simulink model "CyberDog_Motor_FOC_Test"  (R2025b)
settings: Solver=ode4  StartTime=0.0  StopTime=5  FixedStep=0.0001  RelTol=1e-3
InitFcn:
  | p = fileparts(get_param(bdroot,'FileName')); addpath(fullfile(p,'scripts')); motor_params;
undefined symbols (not defined in the file): PolePairs_plant, T_ctrl_mode, T_iq_ref, T_ref_speed, T_TL, Vbus_plant
libraries: mcbplantlib x1, autolibpmsmexterior x1
settings Model: Creator=Baseline  LastModifiedBy=Baseline

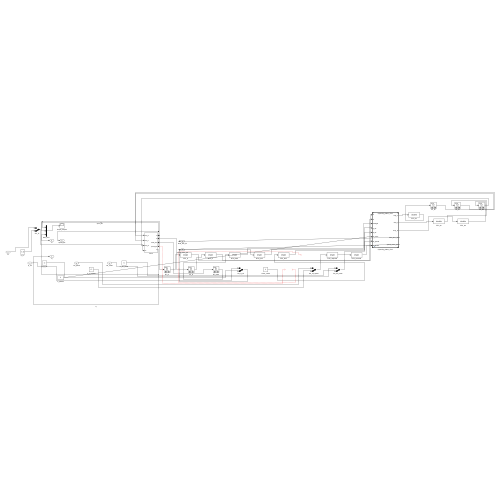
[thumbnail: Simulink's stored preview of the top-level diagram]
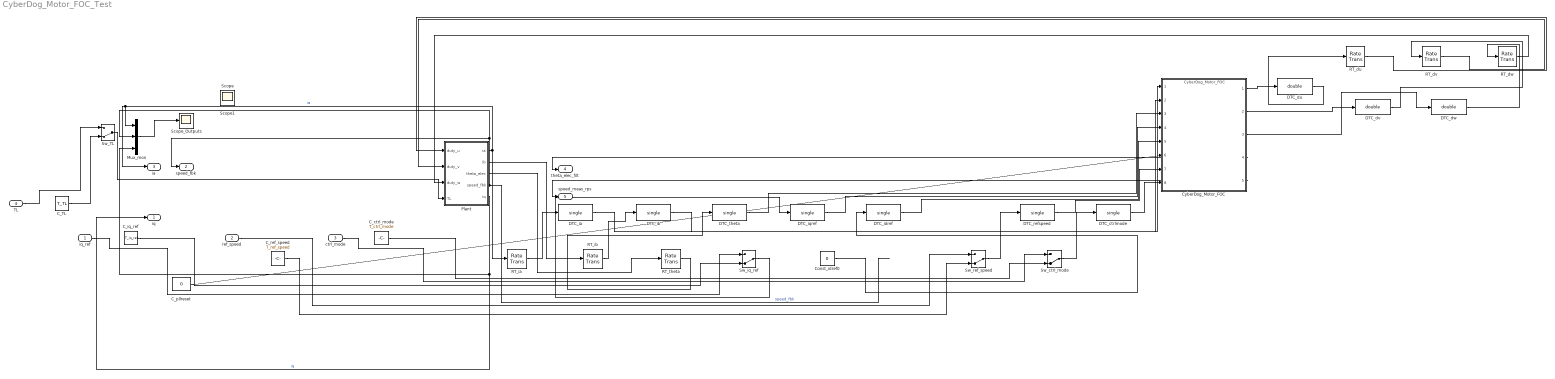
== system CyberDog_Motor_FOC_Test ==
  iq_ref : Inport
  ref_speed : Inport  Port=2
  ctrl_mode : Inport  Port=3
  TL : Inport  Port=4
  C_TL : Constant  Value=T_TL
  C_ctrl_mode : Constant  Value=T_ctrl_mode
  C_iq_ref : Constant  Value=T_iq_ref
  C_pllreset : Constant  Value=0  OutDataTypeStr=single
  C_ref_speed : Constant  Value=T_ref_speed
  Const_idref0 : Constant  Value=0
  CyberDog_Motor_FOC : ModelReference  ModelNameDialog=CyberDog_Motor_FOC  SimulationMode=Normal  ModelReferenceVersion=1.26
  DTC_ctrlmode : DataTypeConversion  OutDataTypeStr=single  SaturateOnIntegerOverflow=off  RndMeth=Floor
  DTC_du : DataTypeConversion  OutDataTypeStr=double  SaturateOnIntegerOverflow=off  RndMeth=Floor
  DTC_dv : DataTypeConversion  OutDataTypeStr=double  SaturateOnIntegerOverflow=off  RndMeth=Floor
  DTC_dw : DataTypeConversion  OutDataTypeStr=double  SaturateOnIntegerOverflow=off  RndMeth=Floor
  DTC_ia : DataTypeConversion  OutDataTypeStr=single  SaturateOnIntegerOverflow=off  RndMeth=Floor
  DTC_ib : DataTypeConversion  OutDataTypeStr=single  SaturateOnIntegerOverflow=off  RndMeth=Floor
  DTC_idref : DataTypeConversion  OutDataTypeStr=single  SaturateOnIntegerOverflow=off  RndMeth=Floor
  DTC_iqref : DataTypeConversion  OutDataTypeStr=single  SaturateOnIntegerOverflow=off  RndMeth=Floor
  DTC_refspeed : DataTypeConversion  OutDataTypeStr=single  SaturateOnIntegerOverflow=off  RndMeth=Floor
  DTC_theta : DataTypeConversion  OutDataTypeStr=single  SaturateOnIntegerOverflow=off  RndMeth=Floor
  Mux_mon : Mux  Inputs=3
  Plant : Subsystem
  RT_du : RateTransition
  RT_dv : RateTransition
  RT_dw : RateTransition
  RT_ia : RateTransition
  RT_ib : RateTransition
  RT_theta : RateTransition
  Scope_Outputs : Scope
      settings: ActiveDisplayYMinimum=-11.406382448656982  ActiveDisplayYMaximum=18.168654247601083
  Sw_TL : ManualSwitch  CurrentSetting=0
  Sw_ctrl_mode : ManualSwitch  CurrentSetting=0
  Sw_iq_ref : ManualSwitch  CurrentSetting=0
  Sw_ref_speed : ManualSwitch  CurrentSetting=0
  iq : Outport
  speed_fbk : Outport  Port=2
  ia : Outport  Port=3
  theta_elec_filt : Outport  Port=4
  speed_meas_rps : Outport  Port=5
  Scope : Scope
      settings: ActiveDisplayYMinimum=-1  ActiveDisplayYMaximum=1
  Scope1 : Scope
      settings: ActiveDisplayYMinimum=-1  ActiveDisplayYMaximum=1
  wires:
  C_TL/1 -> Sw_TL/2
  TL/1 -> Sw_TL/1
  Mux_mon/1 -> Scope_Outputs/1
  Sw_TL/1 -> Plant/4(TL)
  Plant/5(iq) -> iq/1, Mux_mon/3  "iq"
  DTC_dw/1 -> RT_dw/1
  DTC_dv/1 -> RT_dv/1
  DTC_du/1 -> RT_du/1
  DTC_ctrlmode/1 -> CyberDog_Motor_FOC/8
  DTC_refspeed/1 -> CyberDog_Motor_FOC/7
  DTC_idref/1 -> CyberDog_Motor_FOC/5
  DTC_iqref/1 -> CyberDog_Motor_FOC/4
  DTC_theta/1 -> CyberDog_Motor_FOC/3
  DTC_ib/1 -> CyberDog_Motor_FOC/2
  DTC_ia/1 -> CyberDog_Motor_FOC/1
  Sw_ctrl_mode/1 -> DTC_ctrlmode/1
  Sw_ref_speed/1 -> DTC_refspeed/1
  C_ref_speed/1 -> Sw_ref_speed/2
  Sw_iq_ref/1 -> DTC_iqref/1
  C_iq_ref/1 -> Sw_iq_ref/2
  iq_ref/1 -> Sw_iq_ref/1
  CyberDog_Motor_FOC/1 -> DTC_du/1
  CyberDog_Motor_FOC/2 -> DTC_dv/1
  CyberDog_Motor_FOC/3 -> DTC_dw/1
  Plant/1(ia) -> ia/1, Mux_mon/1, RT_ia/1  "ia"
  Plant/2(ib) -> RT_ib/1
  Plant/3(theta_elec) -> RT_theta/1
  Plant/4(speed_fbk) -> Mux_mon/2, speed_fbk/1  "speed_fbk"
  Const_idref0/1 -> DTC_idref/1
  RT_ia/1 -> DTC_ia/1
  RT_ib/1 -> DTC_ib/1
  RT_theta/1 -> DTC_theta/1
  ? -> ?
  RT_du/1 -> Plant/1(duty_u)
  RT_dv/1 -> Plant/2(duty_v)
  RT_dw/1 -> Plant/3(duty_w)
  ctrl_mode/1 -> Sw_ctrl_mode/1
  ref_speed/1 -> Sw_ref_speed/1
  C_ctrl_mode/1 -> Sw_ctrl_mode/2
  C_pllreset/1 -> CyberDog_Motor_FOC/6
  CyberDog_Motor_FOC/4 -> theta_elec_filt/1
  CyberDog_Motor_FOC/5 -> speed_meas_rps/1

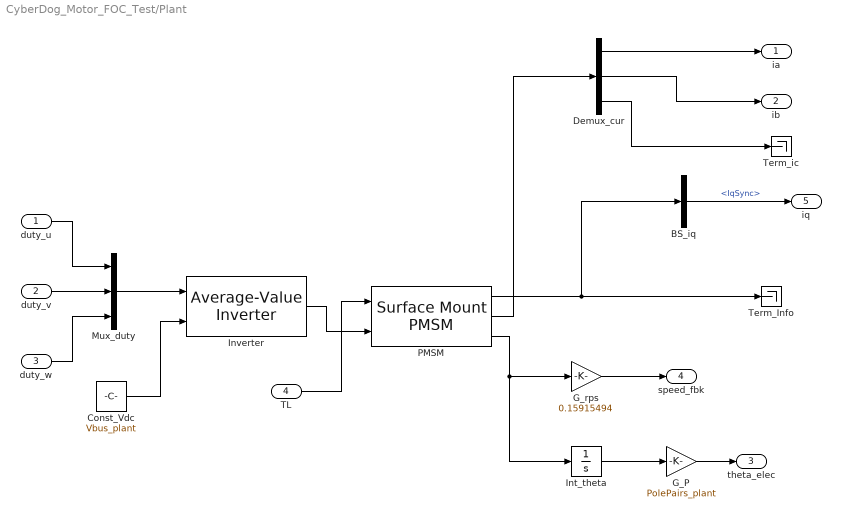
== system CyberDog_Motor_FOC_Test/Plant ==
  duty_u : Inport
  duty_v : Inport  Port=2
  duty_w : Inport  Port=3
  TL : Inport  Port=4
  BS_iq : BusSelector  OutputSignals=IqSync
  Const_Vdc : Constant  Value=Vbus_plant
  Demux_cur : Demux  Outputs=3
  G_P : Gain  Gain=PolePairs_plant
  G_rps : Gain  Gain=0.15915494
  Int_theta : Integrator
  Inverter : mcbplantlib/Average-Value Inverter
      settings: LibrarySourceBlock=mcblib/Electrical Systems/Inverters/Average-Value Inverter
  Mux_duty : Mux  Inputs=3
  PMSM : autolibpmsmexterior/Surface Mount PMSM  port_config=Torque  sim_type=Continuous  Ts=0  P=7  Rs=2.6  Ldq_=2.8e-3  KConstText=Permanent flux linkage constant (lambda_pm):  lambda_pm=0.01  Ke=159.9771  Kt=1.323  mechanical=[0.00015 0.0002 0]  idq0=[0 0]  theta_init=0  omega_init=0  KConst=0.2205  lambda_pm_calc=0.2205  RefBlkName='autolibpmsmexterior/Surface Mount PMSM'  aMode=5  Ldq=[0.0002 0.0002]
  Term_Info : Terminator
  Term_ic : Terminator
  ia : Outport
  ib : Outport  Port=2
  theta_elec : Outport  Port=3
  speed_fbk : Outport  Port=4
  iq : Outport  Port=5
  wires:
  G_rps/1 -> speed_fbk/1
  G_P/1 -> theta_elec/1
  Int_theta/1 -> G_P/1
  Demux_cur/3 -> Term_ic/1
  Demux_cur/1 -> ia/1
  Const_Vdc/1 -> Inverter/2
  Mux_duty/1 -> Inverter/1
  duty_w/1 -> Mux_duty/3
  duty_v/1 -> Mux_duty/2
  duty_u/1 -> Mux_duty/1
  BS_iq/1 -> iq/1  "<IqSync>"
  TL/1 -> PMSM/1
  Inverter/1 -> PMSM/2
  PMSM/1 -> Term_Info/1, BS_iq/1
  PMSM/2 -> Demux_cur/1
  Demux_cur/2 -> ib/1
  PMSM/3 -> G_rps/1, Int_theta/1
